simulink model "Second_Order_Sytsem_P_I_PI_Controller"  (R2024b)
settings: Solver=VariableStepAuto  StartTime=0.0  StopTime=20  RelTol=1e-3
settings Model: Creator=Ahmad  LastModifiedBy=Ahmad

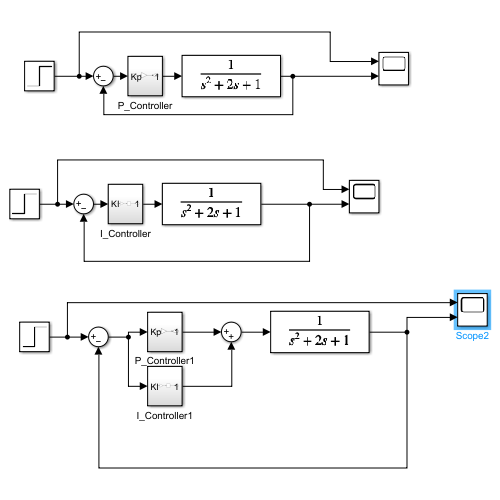
[thumbnail: Simulink's stored preview of the top-level diagram]
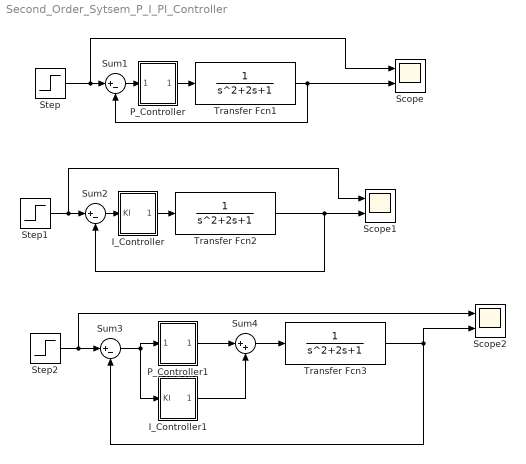
== system Second_Order_Sytsem_P_I_PI_Controller ==
  I_Controller : Subsystem
  I_Controller1 : Subsystem
  P_Controller : Subsystem
  P_Controller1 : Subsystem
  Scope : Scope  NumInputPorts=2
  Scope1 : Scope  NumInputPorts=2
  Scope2 : Scope  NumInputPorts=2
  Step : Step  SampleTime=0
  Step1 : Step  SampleTime=0
  Step2 : Step  SampleTime=0
  Sum1 : Sum  Inputs=|+-
  Sum2 : Sum  Inputs=|+-
  Sum3 : Sum  Inputs=|+-
  Sum4 : Sum  Inputs=|++
  Transfer Fcn1 : TransferFcn
  Transfer Fcn2 : TransferFcn
  Transfer Fcn3 : TransferFcn
  wires:
  Step/1 -> Scope/1, Sum1/1
  Transfer Fcn1/1 -> Sum1/2, Scope/2
  Sum1/1 -> P_Controller/1(Kp)
  P_Controller/1(Out1) -> Transfer Fcn1/1
  I_Controller/1(Out1) -> Transfer Fcn2/1
  Sum2/1 -> I_Controller/1(KI)
  Step1/1 -> Scope1/1, Sum2/1
  Transfer Fcn2/1 -> Sum2/2, Scope1/2
  Step2/1 -> Scope2/1, Sum3/1
  Sum3/1 -> I_Controller1/1(KI), P_Controller1/1(Kp)
  Transfer Fcn3/1 -> Sum3/2, Scope2/2
  P_Controller1/1(Out1) -> Sum4/1
  I_Controller1/1(Out1) -> Sum4/2
  Sum4/1 -> Transfer Fcn3/1

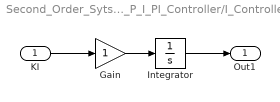
== system Second_Order_Sytsem_P_I_PI_Controller/I_Controller ==
  KI : Inport
  Gain : Gain
  Integrator : Integrator
  Out1 : Outport
  wires:
  KI/1 -> Gain/1
  Gain/1 -> Integrator/1
  Integrator/1 -> Out1/1

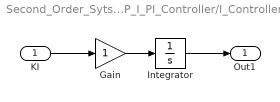
== system Second_Order_Sytsem_P_I_PI_Controller/I_Controller1 ==
  KI : Inport
  Gain : Gain
  Integrator : Integrator
  Out1 : Outport
  wires:
  KI/1 -> Gain/1
  Gain/1 -> Integrator/1
  Integrator/1 -> Out1/1

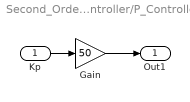
== system Second_Order_Sytsem_P_I_PI_Controller/P_Controller ==
  Kp : Inport
  Gain : Gain  Gain=50
  Out1 : Outport
  wires:
  Gain/1 -> Out1/1
  Kp/1 -> Gain/1

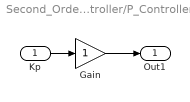
== system Second_Order_Sytsem_P_I_PI_Controller/P_Controller1 ==
  Kp : Inport
  Gain : Gain
  Out1 : Outport
  wires:
  Gain/1 -> Out1/1
  Kp/1 -> Gain/1
